simulink model "case2"  (R2024b)
settings: Solver=FixedStepAuto  StartTime=0  StopTime=1  FixedStep=1e-7  RelTol=1e-3
values from neighbouring files (symbols this model uses):
  SG_D_1_D = 0.01056    [IEEE9_case_parameters.m]    (also in case1_parameters.m; case2_parameters.m; case3_parameters.m; case4_parameters.m)
  SG_D_1_EnableSaturation = 0    [IEEE9_case_parameters.m]    (also in case1_parameters.m; case2_parameters.m; case3_parameters.m; case4_parameters.m)
  SG_D_1_f0 = 60    [IEEE9_case_parameters.m]    (also in case1_parameters.m; case2_parameters.m; case3_parameters.m; case4_parameters.m)
  SG_D_1_H = 7.5    [IEEE9_case_parameters.m]    (also in case1_parameters.m; case2_parameters.m; case3_parameters.m; case4_parameters.m)
  SG_D_1_K_A = 20    [IEEE9_case_parameters.m]    (also in case1_parameters.m; case2_parameters.m; case3_parameters.m; case4_parameters.m)
  SG_D_1_K_E = 1.000000e+1    (= 10)    [IEEE9_case_parameters.m]    (also in case1_parameters.m; case2_parameters.m; case3_parameters.m; case4_parameters.m)
  SG_D_1_K_F = 2.363    [IEEE9_case_parameters.m]    (also in case1_parameters.m; case2_parameters.m; case3_parameters.m; case4_parameters.m)
  SG_D_1_K_s = 0.5    [IEEE9_case_parameters.m]    (also in case1_parameters.m = 5; case2_parameters.m = 5; case3_parameters.m = 5; case4_parameters.m = 5)
  SG_D_1_R_a = 0.001088    [IEEE9_case_parameters.m]    (also in case1_parameters.m; case2_parameters.m; case3_parameters.m; case4_parameters.m)
  SG_D_1_S_A = 1    [IEEE9_case_parameters.m]    (also in case1_parameters.m; case2_parameters.m; case3_parameters.m; case4_parameters.m)
  SG_D_1_S_B = 0.103    [IEEE9_case_parameters.m]    (also in case1_parameters.m; case2_parameters.m; case3_parameters.m; case4_parameters.m)
  SG_D_1_S_N = 10.659857    [IEEE9_case_parameters.m]    (also in case1_parameters.m; case2_parameters.m; case3_parameters.m; case4_parameters.m)
  SG_D_1_SpeedPara = 200    [IEEE9_case_parameters.m]    (also in case1_parameters.m; case2_parameters.m; case3_parameters.m; case4_parameters.m)
  SG_D_1_T_0 = 0.720173    [IEEE9_case_parameters.m]    (also in case1_parameters.m = 0.755522; case2_parameters.m = 0.808931; case3_parameters.m = 0.869402; case4_parameters.m = 0.729316)
  SG_D_1_T_1 = 0.3    [IEEE9_case_parameters.m]    (also in case1_parameters.m; case2_parameters.m; case3_parameters.m; case4_parameters.m)
  SG_D_1_T_2 = 0.05    [IEEE9_case_parameters.m]    (also in case1_parameters.m; case2_parameters.m; case3_parameters.m; case4_parameters.m)
  SG_D_1_T_3 = 0.02    [IEEE9_case_parameters.m]    (also in case1_parameters.m; case2_parameters.m; case3_parameters.m; case4_parameters.m)
  SG_D_1_T_4 = 0.005    [IEEE9_case_parameters.m]    (also in case1_parameters.m; case2_parameters.m; case3_parameters.m; case4_parameters.m)
  SG_D_1_T_A = 0.02    [IEEE9_case_parameters.m]    (also in case1_parameters.m; case2_parameters.m; case3_parameters.m; case4_parameters.m)
  SG_D_1_T_dd = 8.000000e+0    (= 8)    [IEEE9_case_parameters.m]    (also in case1_parameters.m; case2_parameters.m; case3_parameters.m; case4_parameters.m)
  SG_D_1_T_ddd = 0.04    [IEEE9_case_parameters.m]    (also in case1_parameters.m; case2_parameters.m; case3_parameters.m; case4_parameters.m)
  SG_D_1_T_E = 0.314    [IEEE9_case_parameters.m]    (also in case1_parameters.m; case2_parameters.m; case3_parameters.m; case4_parameters.m)
  SG_D_1_T_F = 0.35    [IEEE9_case_parameters.m]    (also in case1_parameters.m; case2_parameters.m; case3_parameters.m; case4_parameters.m)
  SG_D_1_T_qd = 0.8    [IEEE9_case_parameters.m]    (also in case1_parameters.m; case2_parameters.m; case3_parameters.m; case4_parameters.m)
  SG_D_1_T_qdd = 0.02    [IEEE9_case_parameters.m]    (also in case1_parameters.m; case2_parameters.m; case3_parameters.m; case4_parameters.m)
  SG_D_1_T_speed = 0.1    [IEEE9_case_parameters.m]    (also in case1_parameters.m = 200; case2_parameters.m = 200; case3_parameters.m = 200; case4_parameters.m = 200)
  SG_D_1_T_w = 0.5    [IEEE9_case_parameters.m]    (also in case1_parameters.m; case2_parameters.m; case3_parameters.m; case4_parameters.m)
  SG_D_1_V_ref = 1.990276    [IEEE9_case_parameters.m]    (also in case1_parameters.m = 2.042296; case2_parameters.m = 2.051388; case3_parameters.m = 2.089584; case4_parameters.m = 2.01845)
  SG_D_1_w_ref = 376.991118    [IEEE9_case_parameters.m]    (also in case1_parameters.m; case2_parameters.m; case3_parameters.m; case4_parameters.m)
  SG_D_1_wb = 6.000000e+1    (= 60)    [IEEE9_case_parameters.m]    (also in case1_parameters.m; case2_parameters.m; case3_parameters.m; case4_parameters.m)
  SG_D_1_x_d = 1.9    [IEEE9_case_parameters.m]    (also in case1_parameters.m; case2_parameters.m; case3_parameters.m; case4_parameters.m)
  SG_D_1_x_dd = 0.302    [IEEE9_case_parameters.m]    (also in case1_parameters.m; case2_parameters.m; case3_parameters.m; case4_parameters.m)
  SG_D_1_x_ddd = 0.204    [IEEE9_case_parameters.m]    (also in case1_parameters.m; case2_parameters.m; case3_parameters.m; case4_parameters.m)
  SG_D_1_x_l = 0.05    [IEEE9_case_parameters.m]    (also in case1_parameters.m; case2_parameters.m; case3_parameters.m; case4_parameters.m)
  SG_D_1_x_q = 1.3    [IEEE9_case_parameters.m]    (also in case1_parameters.m; case2_parameters.m; case3_parameters.m; case4_parameters.m)
  SG_D_1_x_qd = 0.5    [IEEE9_case_parameters.m]    (also in case1_parameters.m; case2_parameters.m; case3_parameters.m; case4_parameters.m)
  SG_D_1_x_qdd = 0.3    [IEEE9_case_parameters.m]    (also in case1_parameters.m; case2_parameters.m; case3_parameters.m; case4_parameters.m)
  SG_D_2_D = 0.02    [IEEE9_case_parameters.m]    (also in case1_parameters.m; case2_parameters.m; case3_parameters.m; case4_parameters.m)
  SG_D_2_EnableSaturation = 0    [IEEE9_case_parameters.m]    (also in case1_parameters.m; case2_parameters.m; case3_parameters.m; case4_parameters.m)
  SG_D_2_f0 = 60    [IEEE9_case_parameters.m]    (also in case1_parameters.m; case2_parameters.m; case3_parameters.m; case4_parameters.m)
  SG_D_2_H = 8.000000e+0    (= 8)    [IEEE9_case_parameters.m]    (also in case1_parameters.m; case2_parameters.m; case3_parameters.m; case4_parameters.m)
  SG_D_2_K_A = 20    [IEEE9_case_parameters.m]    (also in case1_parameters.m; case2_parameters.m; case3_parameters.m; case4_parameters.m)
  SG_D_2_K_E = 1.000000e+1    (= 10)    [IEEE9_case_parameters.m]    (also in case1_parameters.m; case2_parameters.m; case3_parameters.m; case4_parameters.m)
  SG_D_2_K_F = 2.363    [IEEE9_case_parameters.m]    (also in case1_parameters.m; case2_parameters.m; case3_parameters.m; case4_parameters.m)
  SG_D_2_K_s = 0.5    [IEEE9_case_parameters.m]    (also in case1_parameters.m = 4; case2_parameters.m = 4; case3_parameters.m = 4; case4_parameters.m = 4)
  SG_D_2_R_a = 0.001088    [IEEE9_case_parameters.m]    (also in case1_parameters.m; case2_parameters.m; case3_parameters.m; case4_parameters.m)
  SG_D_2_S_A = 1    [IEEE9_case_parameters.m]    (also in case1_parameters.m; case2_parameters.m; case3_parameters.m; case4_parameters.m)
  SG_D_2_S_B = 0.103    [IEEE9_case_parameters.m]    (also in case1_parameters.m; case2_parameters.m; case3_parameters.m; case4_parameters.m)
  SG_D_2_S_N = 10.659857    [IEEE9_case_parameters.m]    (also in case1_parameters.m; case2_parameters.m; case3_parameters.m; case4_parameters.m)
  SG_D_2_SpeedPara = 200    [IEEE9_case_parameters.m]    (also in case1_parameters.m; case2_parameters.m; case3_parameters.m; case4_parameters.m)
  SG_D_2_T_0 = 1.632913    [IEEE9_case_parameters.m]    (also in case1_parameters.m = 1.632925; case2_parameters.m = 1.632915; case3_parameters.m = 1.632914; case4_parameters.m = 1.632927)
  SG_D_2_T_1 = 0.2    [IEEE9_case_parameters.m]    (also in case1_parameters.m; case2_parameters.m; case3_parameters.m; case4_parameters.m)
  SG_D_2_T_2 = 0.05    [IEEE9_case_parameters.m]    (also in case1_parameters.m; case2_parameters.m; case3_parameters.m; case4_parameters.m)
  SG_D_2_T_3 = 0.02    [IEEE9_case_parameters.m]    (also in case1_parameters.m; case2_parameters.m; case3_parameters.m; case4_parameters.m)
  SG_D_2_T_4 = 0.005    [IEEE9_case_parameters.m]    (also in case1_parameters.m; case2_parameters.m; case3_parameters.m; case4_parameters.m)
  SG_D_2_T_A = 0.02    [IEEE9_case_parameters.m]    (also in case1_parameters.m; case2_parameters.m; case3_parameters.m; case4_parameters.m)
  SG_D_2_T_dd = 7.9    [IEEE9_case_parameters.m]    (also in case1_parameters.m; case2_parameters.m; case3_parameters.m; case4_parameters.m)
  SG_D_2_T_ddd = 0.04    [IEEE9_case_parameters.m]    (also in case1_parameters.m; case2_parameters.m; case3_parameters.m; case4_parameters.m)
  SG_D_2_T_E = 0.314    [IEEE9_case_parameters.m]    (also in case1_parameters.m; case2_parameters.m; case3_parameters.m; case4_parameters.m)
  SG_D_2_T_F = 0.35    [IEEE9_case_parameters.m]    (also in case1_parameters.m; case2_parameters.m; case3_parameters.m; case4_parameters.m)
  SG_D_2_T_qd = 0.8    [IEEE9_case_parameters.m]    (also in case1_parameters.m; case2_parameters.m; case3_parameters.m; case4_parameters.m)
  SG_D_2_T_qdd = 0.015    [IEEE9_case_parameters.m]    (also in case1_parameters.m; case2_parameters.m; case3_parameters.m; case4_parameters.m)
  SG_D_2_T_speed = 0.1    [IEEE9_case_parameters.m]    (also in case1_parameters.m = 150; case2_parameters.m = 150; case3_parameters.m = 150; case4_parameters.m = 150)
  SG_D_2_T_w = 0.35    [IEEE9_case_parameters.m]    (also in case1_parameters.m; case2_parameters.m; case3_parameters.m; case4_parameters.m)
  SG_D_2_V_ref = 2.58547    [IEEE9_case_parameters.m]    (also in case1_parameters.m = 2.597896; case2_parameters.m = 2.587136; case3_parameters.m = 2.586042; case4_parameters.m = 2.599679)
  SG_D_2_w_ref = 376.991118    [IEEE9_case_parameters.m]    (also in case1_parameters.m; case2_parameters.m; case3_parameters.m; case4_parameters.m)
  SG_D_2_wb = 6.000000e+1    (= 60)    [IEEE9_case_parameters.m]    (also in case1_parameters.m; case2_parameters.m; case3_parameters.m; case4_parameters.m)
  SG_D_2_x_d = 1.8    [IEEE9_case_parameters.m]    (also in case1_parameters.m; case2_parameters.m; case3_parameters.m; case4_parameters.m)
  SG_D_2_x_dd = 0.302    [IEEE9_case_parameters.m]    (also in case1_parameters.m; case2_parameters.m; case3_parameters.m; case4_parameters.m)
  SG_D_2_x_ddd = 0.204    [IEEE9_case_parameters.m]    (also in case1_parameters.m; case2_parameters.m; case3_parameters.m; case4_parameters.m)
  SG_D_2_x_l = 0.05    [IEEE9_case_parameters.m]    (also in case1_parameters.m; case2_parameters.m; case3_parameters.m; case4_parameters.m)
  SG_D_2_x_q = 1.25    [IEEE9_case_parameters.m]    (also in case1_parameters.m; case2_parameters.m; case3_parameters.m; case4_parameters.m)
  SG_D_2_x_qd = 0.5    [IEEE9_case_parameters.m]    (also in case1_parameters.m; case2_parameters.m; case3_parameters.m; case4_parameters.m)
  SG_D_2_x_qdd = 0.3    [IEEE9_case_parameters.m]    (also in case1_parameters.m; case2_parameters.m; case3_parameters.m; case4_parameters.m)
  SG_D_3_D = 0.02    [IEEE9_case_parameters.m]    (also in case1_parameters.m; case2_parameters.m; case3_parameters.m; case4_parameters.m)
  SG_D_3_EnableSaturation = 0    [IEEE9_case_parameters.m]    (also in case1_parameters.m; case2_parameters.m; case3_parameters.m; case4_parameters.m)
  SG_D_3_f0 = 60    [IEEE9_case_parameters.m]    (also in case1_parameters.m; case2_parameters.m; case3_parameters.m; case4_parameters.m)
  SG_D_3_H = 7.7    [IEEE9_case_parameters.m]    (also in case1_parameters.m; case2_parameters.m; case3_parameters.m; case4_parameters.m)
  SG_D_3_K_A = 20    [IEEE9_case_parameters.m]    (also in case1_parameters.m; case2_parameters.m; case3_parameters.m; case4_parameters.m)
  SG_D_3_K_E = 1.000000e+1    (= 10)    [IEEE9_case_parameters.m]    (also in case1_parameters.m; case2_parameters.m; case3_parameters.m; case4_parameters.m)
  SG_D_3_K_F = 2.363    [IEEE9_case_parameters.m]    (also in case1_parameters.m; case2_parameters.m; case3_parameters.m; case4_parameters.m)
  SG_D_3_K_s = 0.2    [IEEE9_case_parameters.m]    (also in case1_parameters.m = 2; case2_parameters.m = 2; case3_parameters.m = 2; case4_parameters.m = 2)
  SG_D_3_R_a = 0.001088    [IEEE9_case_parameters.m]    (also in case1_parameters.m; case2_parameters.m; case3_parameters.m; case4_parameters.m)
  SG_D_3_S_A = 1    [IEEE9_case_parameters.m]    (also in case1_parameters.m; case2_parameters.m; case3_parameters.m; case4_parameters.m)
  SG_D_3_S_B = 0.103    [IEEE9_case_parameters.m]    (also in case1_parameters.m; case2_parameters.m; case3_parameters.m; case4_parameters.m)
  SG_D_3_S_N = 10.659857    [IEEE9_case_parameters.m]    (also in case1_parameters.m; case2_parameters.m; case3_parameters.m; case4_parameters.m)
  SG_D_3_SpeedPara = 200    [IEEE9_case_parameters.m]    (also in case1_parameters.m; case2_parameters.m; case3_parameters.m; case4_parameters.m)
  SG_D_3_T_0 = 0.850788    [IEEE9_case_parameters.m]    (also in case1_parameters.m = 0.850786; case2_parameters.m = 0.850787; case3_parameters.m; case4_parameters.m = 0.850786)
  SG_D_3_T_1 = 0.2    [IEEE9_case_parameters.m]    (also in case1_parameters.m; case2_parameters.m; case3_parameters.m; case4_parameters.m)
  SG_D_3_T_2 = 0.05    [IEEE9_case_parameters.m]    (also in case1_parameters.m; case2_parameters.m; case3_parameters.m; case4_parameters.m)
  SG_D_3_T_3 = 0.02    [IEEE9_case_parameters.m]    (also in case1_parameters.m; case2_parameters.m; case3_parameters.m; case4_parameters.m)
  SG_D_3_T_4 = 0.005    [IEEE9_case_parameters.m]    (also in case1_parameters.m; case2_parameters.m; case3_parameters.m; case4_parameters.m)
  SG_D_3_T_A = 0.02    [IEEE9_case_parameters.m]    (also in case1_parameters.m; case2_parameters.m; case3_parameters.m; case4_parameters.m)
  SG_D_3_T_dd = 8.1    [IEEE9_case_parameters.m]    (also in case1_parameters.m; case2_parameters.m; case3_parameters.m; case4_parameters.m)
  SG_D_3_T_ddd = 0.04    [IEEE9_case_parameters.m]    (also in case1_parameters.m; case2_parameters.m; case3_parameters.m; case4_parameters.m)
  SG_D_3_T_E = 0.314    [IEEE9_case_parameters.m]    (also in case1_parameters.m; case2_parameters.m; case3_parameters.m; case4_parameters.m)
  SG_D_3_T_F = 0.35    [IEEE9_case_parameters.m]    (also in case1_parameters.m; case2_parameters.m; case3_parameters.m; case4_parameters.m)
  SG_D_3_T_qd = 0.8    [IEEE9_case_parameters.m]    (also in case1_parameters.m; case2_parameters.m; case3_parameters.m; case4_parameters.m)
  SG_D_3_T_qdd = 0.015    [IEEE9_case_parameters.m]    (also in case1_parameters.m; case2_parameters.m; case3_parameters.m; case4_parameters.m)
  SG_D_3_T_speed = 0.1    [IEEE9_case_parameters.m]    (also in case1_parameters.m = 180; case2_parameters.m = 180; case3_parameters.m = 180; case4_parameters.m = 180)
  SG_D_3_T_w = 0.4    [IEEE9_case_parameters.m]    (also in case1_parameters.m; case2_parameters.m; case3_parameters.m; case4_parameters.m)
  SG_D_3_V_ref = 1.892727    [IEEE9_case_parameters.m]    (also in case1_parameters.m = 1.906439; case2_parameters.m = 1.895535; case3_parameters.m = 1.892105; case4_parameters.m = 1.906598)
  SG_D_3_w_ref = 376.991118    [IEEE9_case_parameters.m]    (also in case1_parameters.m; case2_parameters.m; case3_parameters.m; case4_parameters.m)
  SG_D_3_wb = 6.000000e+1    (= 60)    [IEEE9_case_parameters.m]    (also in case1_parameters.m; case2_parameters.m; case3_parameters.m; case4_parameters.m)
  SG_D_3_x_d = 1.85    [IEEE9_case_parameters.m]    (also in case1_parameters.m; case2_parameters.m; case3_parameters.m; case4_parameters.m)
  SG_D_3_x_dd = 0.302    [IEEE9_case_parameters.m]    (also in case1_parameters.m; case2_parameters.m; case3_parameters.m; case4_parameters.m)
  SG_D_3_x_ddd = 0.204    [IEEE9_case_parameters.m]    (also in case1_parameters.m; case2_parameters.m; case3_parameters.m; case4_parameters.m)
  SG_D_3_x_l = 0.05    [IEEE9_case_parameters.m]    (also in case1_parameters.m; case2_parameters.m; case3_parameters.m; case4_parameters.m)
  SG_D_3_x_q = 1.2    [IEEE9_case_parameters.m]    (also in case1_parameters.m; case2_parameters.m; case3_parameters.m; case4_parameters.m)
  SG_D_3_x_qd = 0.5    [IEEE9_case_parameters.m]    (also in case1_parameters.m; case2_parameters.m; case3_parameters.m; case4_parameters.m)
  SG_D_3_x_qdd = 0.3    [IEEE9_case_parameters.m]    (also in case1_parameters.m; case2_parameters.m; case3_parameters.m; case4_parameters.m)
(part 2 of 12)

== system case2/SG_D_2 ==
  v_d_SG_D_2 : Inport
  v_q_SG_D_2 : Inport  Port=2
  E_fd_SG_D_2 : Integrator  InitialCondition=3.174272760835506
  Px_1_SG_D_2 : Integrator  InitialCondition=0.0
  Px_2_SG_D_2 : Integrator  InitialCondition=0.0
  Px_3_SG_D_2 : Integrator  InitialCondition=1.5518206865207427e-24
  R_f_SG_D_2 : Integrator  InitialCondition=21.43087581101229
  T_e_SG_D_2_block : Subsystem
  T_m_SG_D_2 : Integrator  InitialCondition=1.6329149167652506
  V_f_SG_D_2 : Integrator  InitialCondition=31.742727608355057
  d_E_fd_SG_D_2_block : Subsystem
  d_Px_1_SG_D_2_block : Subsystem
  d_Px_2_SG_D_2_block : Subsystem
  d_Px_3_SG_D_2_block : Subsystem
  d_R_f_SG_D_2_block : Subsystem
  d_T_m_SG_D_2_block : Subsystem
  d_V_f_SG_D_2_block : Subsystem
  d_psi_1d_SG_D_2_block : Subsystem
  d_psi_d_SG_D_2_block : Subsystem
  d_psi_fd_SG_D_2_block : Subsystem
  d_psi_gq_SG_D_2_block : Subsystem
  d_psi_kq_SG_D_2_block : Subsystem
  d_psi_q_SG_D_2_block : Subsystem
  d_theta_SG_D_2_block : Subsystem
  d_w_SG_D_2_block : Subsystem
  i_d_SG_D_2_block : Subsystem
  i_q_SG_D_2_block : Subsystem
  psi_1d_SG_D_2 : Integrator  InitialCondition=0.5787158687798319
  psi_d_SG_D_2 : Integrator  InitialCondition=0.504557100435384
  psi_fd_SG_D_2 : Integrator  InitialCondition=0.9524760612358489
  psi_gq_SG_D_2 : Integrator  InitialCondition=0.5192590741580433
  psi_kq_SG_D_2 : Integrator  InitialCondition=-0.8308145186528693
  psi_q_SG_D_2 : Integrator  InitialCondition=-0.8654317902634056
  theta_SG_D_2 : Integrator  InitialCondition=1.1962684178296192
  theta_SG_D_2_out_block : Subsystem
  w_SG_D_2 : Integrator  InitialCondition=376.99111843077515
  w_SG_D_2_out_block : Subsystem
  i_d_SG_D_2 : Outport
  i_q_SG_D_2 : Outport  Port=2
  T_e_SG_D_2 : Outport  Port=3
  w_SG_D_2_out : Outport  Port=4
  theta_SG_D_2_out : Outport  Port=5
  wires:
  d_T_m_SG_D_2_block/1(Blockout_d_T_m_SG_D_2_4b089) -> T_m_SG_D_2/1
  T_e_SG_D_2_block/1(Blockout_T_e_SG_D_2_b8deb) -> T_e_SG_D_2/1
  d_Px_2_SG_D_2_block/1(Blockout_d_Px_2_SG_D_2_22689) -> Px_2_SG_D_2/1
  w_SG_D_2/1 -> d_psi_d_SG_D_2_block/9(State_w_SG_D_2_e892d), d_w_SG_D_2_block/1(State_w_SG_D_2_a0af8), d_V_f_SG_D_2_block/13(State_w_SG_D_2_f97cf), d_psi_q_SG_D_2_block/9(State_w_SG_D_2_c2d17), d_V_f_SG_D_2_block/8(State_w_SG_D_2_9712b), d_theta_SG_D_2_block/1(State_w_SG_D_2_08923), d_Px_2_SG_D_2_block/4(State_w_SG_D_2_45781), d_Px_3_SG_D_2_block/6(State_w_SG_D_2_38541), d_Px_1_SG_D_2_block/2(State_w_SG_D_2_84017), w_SG_D_2_out_block/1(State_w_SG_D_2_b0f95), d_T_m_SG_D_2_block/1(State_w_SG_D_2_14e8c)
  d_theta_SG_D_2_block/1(Blockout_d_theta_SG_D_2_633fd) -> theta_SG_D_2/1
  d_Px_1_SG_D_2_block/1(Blockout_d_Px_1_SG_D_2_b8a6d) -> Px_1_SG_D_2/1
  psi_q_SG_D_2/1 -> d_psi_d_SG_D_2_block/8(State_psi_q_SG_D_2_fe7e7), d_psi_q_SG_D_2_block/3(State_psi_q_SG_D_2_bc55a), d_psi_gq_SG_D_2_block/6(State_psi_q_SG_D_2_40973), d_psi_gq_SG_D_2_block/9(State_psi_q_SG_D_2_4a342), d_psi_kq_SG_D_2_block/5(State_psi_q_SG_D_2_76d71), d_w_SG_D_2_block/7(State_psi_q_SG_D_2_3518a), d_V_f_SG_D_2_block/7(State_psi_q_SG_D_2_f4c0e), d_w_SG_D_2_block/6(State_psi_q_SG_D_2_c02e1), d_V_f_SG_D_2_block/11(State_psi_q_SG_D_2_6c1aa), i_q_SG_D_2_block/3(State_psi_q_SG_D_2_d1f7c), i_d_SG_D_2_block/3(State_psi_q_SG_D_2_74918), T_e_SG_D_2_block/4(State_psi_q_SG_D_2_d45b5), T_e_SG_D_2_block/5(State_psi_q_SG_D_2_80989)
  w_SG_D_2_out_block/1(Blockout_w_SG_D_2_out_f6fd7) -> w_SG_D_2_out/1
  psi_fd_SG_D_2/1 -> d_psi_fd_SG_D_2_block/2(State_psi_fd_SG_D_2_9a5f7), d_psi_fd_SG_D_2_block/4(State_psi_fd_SG_D_2_7d5d1), d_psi_1d_SG_D_2_block/2(State_psi_fd_SG_D_2_21e47), d_V_f_SG_D_2_block/6(State_psi_fd_SG_D_2_145b7), d_w_SG_D_2_block/10(State_psi_fd_SG_D_2_89ccd), T_e_SG_D_2_block/8(State_psi_fd_SG_D_2_cd007), d_psi_fd_SG_D_2_block/7(State_psi_fd_SG_D_2_aa5d6), i_q_SG_D_2_block/7(State_psi_fd_SG_D_2_212cc), i_d_SG_D_2_block/7(State_psi_fd_SG_D_2_463f2), d_psi_1d_SG_D_2_block/5(State_psi_fd_SG_D_2_221ae), d_psi_d_SG_D_2_block/3(State_psi_fd_SG_D_2_19126), d_psi_fd_SG_D_2_block/10(State_psi_fd_SG_D_2_e8112)
  d_Px_3_SG_D_2_block/1(Blockout_d_Px_3_SG_D_2_0a542) -> Px_3_SG_D_2/1
  v_d_SG_D_2/1 -> d_psi_d_SG_D_2_block/4(Input_v_d_SG_D_2_3ae72), d_psi_q_SG_D_2_block/4(Input_v_d_SG_D_2_0f316)
  d_V_f_SG_D_2_block/1(Blockout_d_V_f_SG_D_2_fa732) -> V_f_SG_D_2/1
  v_q_SG_D_2/1 -> d_psi_d_SG_D_2_block/6(Input_v_q_SG_D_2_cabf7), d_psi_q_SG_D_2_block/6(Input_v_q_SG_D_2_6312d)
  theta_SG_D_2/1 -> i_d_SG_D_2_block/4(State_theta_SG_D_2_67c6e), d_psi_q_SG_D_2_block/5(State_theta_SG_D_2_f78f2), d_psi_d_SG_D_2_block/7(State_theta_SG_D_2_a0973), i_d_SG_D_2_block/8(State_theta_SG_D_2_e4d3c), d_psi_d_SG_D_2_block/5(State_theta_SG_D_2_01400), d_psi_q_SG_D_2_block/7(State_theta_SG_D_2_25da5), i_q_SG_D_2_block/8(State_theta_SG_D_2_6d11f), theta_SG_D_2_out_block/1(State_theta_SG_D_2_6b056), i_q_SG_D_2_block/4(State_theta_SG_D_2_14f06)
  Px_2_SG_D_2/1 -> d_Px_3_SG_D_2_block/2(State_Px_2_SG_D_2_61639), d_Px_3_SG_D_2_block/3(State_Px_2_SG_D_2_4e1b7), d_Px_2_SG_D_2_block/1(State_Px_2_SG_D_2_f980a)
  psi_gq_SG_D_2/1 -> d_psi_q_SG_D_2_block/1(State_psi_gq_SG_D_2_02402), d_psi_gq_SG_D_2_block/1(State_psi_gq_SG_D_2_a2a06), d_psi_gq_SG_D_2_block/2(State_psi_gq_SG_D_2_83ab1), d_psi_gq_SG_D_2_block/4(State_psi_gq_SG_D_2_c1c72), d_psi_kq_SG_D_2_block/1(State_psi_gq_SG_D_2_2ecc4), d_psi_kq_SG_D_2_block/3(State_psi_gq_SG_D_2_6238c), d_V_f_SG_D_2_block/9(State_psi_gq_SG_D_2_6385a), d_psi_gq_SG_D_2_block/7(State_psi_gq_SG_D_2_7b31f), i_q_SG_D_2_block/1(State_psi_gq_SG_D_2_62065), d_w_SG_D_2_block/4(State_psi_gq_SG_D_2_fa13f), T_e_SG_D_2_block/2(State_psi_gq_SG_D_2_708b9), i_d_SG_D_2_block/1(State_psi_gq_SG_D_2_419a5)
  psi_1d_SG_D_2/1 -> d_psi_fd_SG_D_2_block/3(State_psi_1d_SG_D_2_9e249), d_psi_fd_SG_D_2_block/8(State_psi_1d_SG_D_2_c9b22), d_psi_fd_SG_D_2_block/5(State_psi_1d_SG_D_2_19e55), d_psi_d_SG_D_2_block/1(State_psi_1d_SG_D_2_3fdee), d_psi_1d_SG_D_2_block/1(State_psi_1d_SG_D_2_7ee43), d_psi_1d_SG_D_2_block/3(State_psi_1d_SG_D_2_6e6f3), d_w_SG_D_2_block/8(State_psi_1d_SG_D_2_8aa3a), d_V_f_SG_D_2_block/4(State_psi_1d_SG_D_2_c0128), i_d_SG_D_2_block/5(State_psi_1d_SG_D_2_37338), i_q_SG_D_2_block/5(State_psi_1d_SG_D_2_3e03a), T_e_SG_D_2_block/6(State_psi_1d_SG_D_2_98cfc)
  T_m_SG_D_2/1 -> d_T_m_SG_D_2_block/2(State_T_m_SG_D_2_165ac), d_w_SG_D_2_block/2(State_T_m_SG_D_2_deb70)
  Px_1_SG_D_2/1 -> d_Px_1_SG_D_2_block/1(State_Px_1_SG_D_2_d590c), d_Px_3_SG_D_2_block/4(State_Px_1_SG_D_2_cef04), d_Px_3_SG_D_2_block/5(State_Px_1_SG_D_2_2a306), d_Px_2_SG_D_2_block/3(State_Px_1_SG_D_2_9c84f), d_Px_2_SG_D_2_block/2(State_Px_1_SG_D_2_3257e)
  i_d_SG_D_2_block/1(Blockout_i_d_SG_D_2_4df8b) -> i_d_SG_D_2/1
  psi_d_SG_D_2/1 -> d_psi_fd_SG_D_2_block/6(State_psi_d_SG_D_2_bc679), d_psi_fd_SG_D_2_block/9(State_psi_d_SG_D_2_749a1), d_psi_d_SG_D_2_block/2(State_psi_d_SG_D_2_d60ed), d_psi_q_SG_D_2_block/8(State_psi_d_SG_D_2_afeb6), d_psi_1d_SG_D_2_block/4(State_psi_d_SG_D_2_2e599), d_w_SG_D_2_block/3(State_psi_d_SG_D_2_6bbdf), d_V_f_SG_D_2_block/12(State_psi_d_SG_D_2_bc1e6), i_d_SG_D_2_block/6(State_psi_d_SG_D_2_8c17d), i_q_SG_D_2_block/6(State_psi_d_SG_D_2_1a46c), d_w_SG_D_2_block/9(State_psi_d_SG_D_2_a921b), T_e_SG_D_2_block/1(State_psi_d_SG_D_2_1b998), T_e_SG_D_2_block/7(State_psi_d_SG_D_2_92f27), d_V_f_SG_D_2_block/5(State_psi_d_SG_D_2_b5e07)
  psi_kq_SG_D_2/1 -> d_psi_q_SG_D_2_block/2(State_psi_kq_SG_D_2_3ae4e), d_psi_gq_SG_D_2_block/5(State_psi_kq_SG_D_2_816be), d_psi_kq_SG_D_2_block/2(State_psi_kq_SG_D_2_ff9b7), d_psi_kq_SG_D_2_block/4(State_psi_kq_SG_D_2_b8096), d_w_SG_D_2_block/5(State_psi_kq_SG_D_2_e86be), d_V_f_SG_D_2_block/10(State_psi_kq_SG_D_2_aa54e), i_q_SG_D_2_block/2(State_psi_kq_SG_D_2_46994), T_e_SG_D_2_block/3(State_psi_kq_SG_D_2_15175), d_psi_gq_SG_D_2_block/3(State_psi_kq_SG_D_2_ccf89), i_d_SG_D_2_block/2(State_psi_kq_SG_D_2_2885e), d_psi_gq_SG_D_2_block/8(State_psi_kq_SG_D_2_a9de5)
  d_psi_1d_SG_D_2_block/1(Blockout_d_psi_1d_SG_D_2_52177) -> psi_1d_SG_D_2/1
  d_psi_q_SG_D_2_block/1(Blockout_d_psi_q_SG_D_2_71529) -> psi_q_SG_D_2/1
  d_psi_d_SG_D_2_block/1(Blockout_d_psi_d_SG_D_2_b24b5) -> psi_d_SG_D_2/1
  d_psi_kq_SG_D_2_block/1(Blockout_d_psi_kq_SG_D_2_e0637) -> psi_kq_SG_D_2/1
  i_q_SG_D_2_block/1(Blockout_i_q_SG_D_2_bbd87) -> i_q_SG_D_2/1
  R_f_SG_D_2/1 -> d_R_f_SG_D_2_block/2(State_R_f_SG_D_2_5b4f1), d_V_f_SG_D_2_block/2(State_R_f_SG_D_2_7d620)
  theta_SG_D_2_out_block/1(Blockout_theta_SG_D_2_out_ba39c) -> theta_SG_D_2_out/1
  d_w_SG_D_2_block/1(Blockout_d_w_SG_D_2_da6a7) -> w_SG_D_2/1
  d_psi_gq_SG_D_2_block/1(Blockout_d_psi_gq_SG_D_2_be7cc) -> psi_gq_SG_D_2/1
  d_R_f_SG_D_2_block/1(Blockout_d_R_f_SG_D_2_fdb54) -> R_f_SG_D_2/1
  V_f_SG_D_2/1 -> d_V_f_SG_D_2_block/14(State_V_f_SG_D_2_2e53e), d_E_fd_SG_D_2_block/2(State_V_f_SG_D_2_edff6)
  Px_3_SG_D_2/1 -> d_Px_3_SG_D_2_block/1(State_Px_3_SG_D_2_650ae), d_V_f_SG_D_2_block/3(State_Px_3_SG_D_2_fb941)
  d_E_fd_SG_D_2_block/1(Blockout_d_E_fd_SG_D_2_d404e) -> E_fd_SG_D_2/1
  E_fd_SG_D_2/1 -> d_V_f_SG_D_2_block/1(State_E_fd_SG_D_2_39bcd), d_R_f_SG_D_2_block/1(State_E_fd_SG_D_2_001ad), d_E_fd_SG_D_2_block/1(State_E_fd_SG_D_2_04f17), d_psi_fd_SG_D_2_block/1(State_E_fd_SG_D_2_538cb)
  d_psi_fd_SG_D_2_block/1(Blockout_d_psi_fd_SG_D_2_3c09c) -> psi_fd_SG_D_2/1

== system case2/SG_D_3 ==
  v_d_SG_D_3 : Inport
  v_q_SG_D_3 : Inport  Port=2
  E_fd_SG_D_3 : Integrator  InitialCondition=1.7910701006182943
  Px_1_SG_D_3 : Integrator  InitialCondition=0.0
  Px_2_SG_D_3 : Integrator  InitialCondition=0.0
  Px_3_SG_D_3 : Integrator  InitialCondition=-1.0387374102072241e-24
  R_f_SG_D_3 : Integrator  InitialCondition=12.092281850745799
  T_e_SG_D_3_block : Subsystem
  T_m_SG_D_3 : Integrator  InitialCondition=0.8507871254664061
  V_f_SG_D_3 : Integrator  InitialCondition=17.910701006182943
  d_E_fd_SG_D_3_block : Subsystem
  d_Px_1_SG_D_3_block : Subsystem
  d_Px_2_SG_D_3_block : Subsystem
  d_Px_3_SG_D_3_block : Subsystem
  d_R_f_SG_D_3_block : Subsystem
  d_T_m_SG_D_3_block : Subsystem
  d_V_f_SG_D_3_block : Subsystem
  d_psi_1d_SG_D_3_block : Subsystem
  d_psi_d_SG_D_3_block : Subsystem
  d_psi_fd_SG_D_3_block : Subsystem
  d_psi_gq_SG_D_3_block : Subsystem
  d_psi_kq_SG_D_3_block : Subsystem
  d_psi_q_SG_D_3_block : Subsystem
  d_theta_SG_D_3_block : Subsystem
  d_w_SG_D_3_block : Subsystem
  i_d_SG_D_3_block : Subsystem
  i_q_SG_D_3_block : Subsystem
  psi_1d_SG_D_3 : Integrator  InitialCondition=0.7172513618057285
  psi_d_SG_D_3 : Integrator  InitialCondition=0.6874230635053793
  psi_fd_SG_D_3 : Integrator  InitialCondition=0.8675859852394877
  psi_gq_SG_D_3 : Integrator  InitialCondition=0.42439253500886276
  psi_kq_SG_D_3 : Integrator  InitialCondition=-0.6972163075145603
  psi_q_SG_D_3 : Integrator  InitialCondition=-0.7275300600151934
  theta_SG_D_3 : Integrator  InitialCondition=0.8839403378010618
  theta_SG_D_3_out_block : Subsystem
  w_SG_D_3 : Integrator  InitialCondition=376.99111843077515
  w_SG_D_3_out_block : Subsystem
  i_d_SG_D_3 : Outport
  i_q_SG_D_3 : Outport  Port=2
  T_e_SG_D_3 : Outport  Port=3
  w_SG_D_3_out : Outport  Port=4
  theta_SG_D_3_out : Outport  Port=5
  wires:
  d_Px_1_SG_D_3_block/1(Blockout_d_Px_1_SG_D_3_ecaac) -> Px_1_SG_D_3/1
  w_SG_D_3/1 -> d_psi_q_SG_D_3_block/9(State_w_SG_D_3_6302a), d_psi_d_SG_D_3_block/9(State_w_SG_D_3_819b4), d_w_SG_D_3_block/1(State_w_SG_D_3_97bb8), d_V_f_SG_D_3_block/8(State_w_SG_D_3_a95f7), d_V_f_SG_D_3_block/13(State_w_SG_D_3_43b52), d_theta_SG_D_3_block/1(State_w_SG_D_3_3d54c), d_T_m_SG_D_3_block/1(State_w_SG_D_3_ad955), d_Px_1_SG_D_3_block/2(State_w_SG_D_3_fb455), d_Px_3_SG_D_3_block/6(State_w_SG_D_3_a9ec3), d_Px_2_SG_D_3_block/4(State_w_SG_D_3_9f660), w_SG_D_3_out_block/1(State_w_SG_D_3_99a7f)
  R_f_SG_D_3/1 -> d_V_f_SG_D_3_block/2(State_R_f_SG_D_3_88428), d_R_f_SG_D_3_block/2(State_R_f_SG_D_3_e823d)
  w_SG_D_3_out_block/1(Blockout_w_SG_D_3_out_0217d) -> w_SG_D_3_out/1
  d_Px_2_SG_D_3_block/1(Blockout_d_Px_2_SG_D_3_b7721) -> Px_2_SG_D_3/1
  d_w_SG_D_3_block/1(Blockout_d_w_SG_D_3_1b2eb) -> w_SG_D_3/1
  Px_1_SG_D_3/1 -> d_Px_1_SG_D_3_block/1(State_Px_1_SG_D_3_6a762), d_Px_3_SG_D_3_block/4(State_Px_1_SG_D_3_dfdda), d_Px_2_SG_D_3_block/3(State_Px_1_SG_D_3_de3ab), d_Px_3_SG_D_3_block/5(State_Px_1_SG_D_3_46ef9), d_Px_2_SG_D_3_block/2(State_Px_1_SG_D_3_07a77)
  d_theta_SG_D_3_block/1(Blockout_d_theta_SG_D_3_7f2c9) -> theta_SG_D_3/1
  d_T_m_SG_D_3_block/1(Blockout_d_T_m_SG_D_3_4be0a) -> T_m_SG_D_3/1
  psi_fd_SG_D_3/1 -> d_psi_fd_SG_D_3_block/2(State_psi_fd_SG_D_3_11ef0), d_psi_fd_SG_D_3_block/4(State_psi_fd_SG_D_3_d3ee5), d_psi_fd_SG_D_3_block/7(State_psi_fd_SG_D_3_7f5a7), d_psi_fd_SG_D_3_block/10(State_psi_fd_SG_D_3_791d9), d_psi_d_SG_D_3_block/3(State_psi_fd_SG_D_3_c348d), d_psi_1d_SG_D_3_block/2(State_psi_fd_SG_D_3_ea669), d_psi_1d_SG_D_3_block/5(State_psi_fd_SG_D_3_4d32c), d_w_SG_D_3_block/10(State_psi_fd_SG_D_3_99c58), d_V_f_SG_D_3_block/6(State_psi_fd_SG_D_3_9c647), i_d_SG_D_3_block/7(State_psi_fd_SG_D_3_d8144), T_e_SG_D_3_block/8(State_psi_fd_SG_D_3_e25ec), i_q_SG_D_3_block/7(State_psi_fd_SG_D_3_16b63)
  d_Px_3_SG_D_3_block/1(Blockout_d_Px_3_SG_D_3_317cb) -> Px_3_SG_D_3/1
  v_d_SG_D_3/1 -> d_psi_d_SG_D_3_block/4(Input_v_d_SG_D_3_4a6e0), d_psi_q_SG_D_3_block/4(Input_v_d_SG_D_3_18c9f)
  v_q_SG_D_3/1 -> d_psi_q_SG_D_3_block/6(Input_v_q_SG_D_3_33c03), d_psi_d_SG_D_3_block/6(Input_v_q_SG_D_3_b307b)
  theta_SG_D_3/1 -> d_psi_d_SG_D_3_block/5(State_theta_SG_D_3_26889), i_q_SG_D_3_block/4(State_theta_SG_D_3_d6326), i_d_SG_D_3_block/4(State_theta_SG_D_3_a77c5), i_d_SG_D_3_block/8(State_theta_SG_D_3_da351), d_psi_q_SG_D_3_block/7(State_theta_SG_D_3_49b48), d_psi_d_SG_D_3_block/7(State_theta_SG_D_3_a755b), i_q_SG_D_3_block/8(State_theta_SG_D_3_67ddf), theta_SG_D_3_out_block/1(State_theta_SG_D_3_32087), d_psi_q_SG_D_3_block/5(State_theta_SG_D_3_06d3e)
  psi_gq_SG_D_3/1 -> d_psi_q_SG_D_3_block/1(State_psi_gq_SG_D_3_520bc), d_psi_gq_SG_D_3_block/4(State_psi_gq_SG_D_3_a44eb), d_psi_gq_SG_D_3_block/1(State_psi_gq_SG_D_3_621ad), d_w_SG_D_3_block/4(State_psi_gq_SG_D_3_6c331), d_psi_gq_SG_D_3_block/7(State_psi_gq_SG_D_3_1d830), d_V_f_SG_D_3_block/9(State_psi_gq_SG_D_3_26e2a), i_d_SG_D_3_block/1(State_psi_gq_SG_D_3_d77e8), d_psi_gq_SG_D_3_block/2(State_psi_gq_SG_D_3_3b232), d_psi_kq_SG_D_3_block/1(State_psi_gq_SG_D_3_a1641), i_q_SG_D_3_block/1(State_psi_gq_SG_D_3_6f435), T_e_SG_D_3_block/2(State_psi_gq_SG_D_3_f5567), d_psi_kq_SG_D_3_block/3(State_psi_gq_SG_D_3_25fe6)
  Px_2_SG_D_3/1 -> d_Px_3_SG_D_3_block/2(State_Px_2_SG_D_3_6ab48), d_Px_2_SG_D_3_block/1(State_Px_2_SG_D_3_e4ce9), d_Px_3_SG_D_3_block/3(State_Px_2_SG_D_3_b9577)
  psi_q_SG_D_3/1 -> d_psi_q_SG_D_3_block/3(State_psi_q_SG_D_3_df188), d_psi_gq_SG_D_3_block/6(State_psi_q_SG_D_3_1c866), d_psi_kq_SG_D_3_block/5(State_psi_q_SG_D_3_91d06), d_w_SG_D_3_block/6(State_psi_q_SG_D_3_be05f), d_psi_d_SG_D_3_block/8(State_psi_q_SG_D_3_2a9ae), d_V_f_SG_D_3_block/7(State_psi_q_SG_D_3_7abe7), i_d_SG_D_3_block/3(State_psi_q_SG_D_3_0448a), T_e_SG_D_3_block/4(State_psi_q_SG_D_3_e157f), d_w_SG_D_3_block/7(State_psi_q_SG_D_3_3cf4a), i_q_SG_D_3_block/3(State_psi_q_SG_D_3_d128a), d_psi_gq_SG_D_3_block/9(State_psi_q_SG_D_3_e7378), d_V_f_SG_D_3_block/11(State_psi_q_SG_D_3_24c47), T_e_SG_D_3_block/5(State_psi_q_SG_D_3_b3ce3)
  psi_d_SG_D_3/1 -> d_psi_fd_SG_D_3_block/6(State_psi_d_SG_D_3_b2294), d_psi_fd_SG_D_3_block/9(State_psi_d_SG_D_3_a29f0), d_psi_d_SG_D_3_block/2(State_psi_d_SG_D_3_921ca), d_psi_q_SG_D_3_block/8(State_psi_d_SG_D_3_6d66b), d_psi_1d_SG_D_3_block/4(State_psi_d_SG_D_3_a70b8), d_V_f_SG_D_3_block/5(State_psi_d_SG_D_3_0d4e4), d_V_f_SG_D_3_block/12(State_psi_d_SG_D_3_c49cc), d_w_SG_D_3_block/9(State_psi_d_SG_D_3_7b9ed), d_w_SG_D_3_block/3(State_psi_d_SG_D_3_3a32b), i_d_SG_D_3_block/6(State_psi_d_SG_D_3_23dc4), i_q_SG_D_3_block/6(State_psi_d_SG_D_3_56c73), T_e_SG_D_3_block/1(State_psi_d_SG_D_3_e6750), T_e_SG_D_3_block/7(State_psi_d_SG_D_3_a51a8)
  psi_kq_SG_D_3/1 -> d_psi_q_SG_D_3_block/2(State_psi_kq_SG_D_3_0e323), d_psi_gq_SG_D_3_block/3(State_psi_kq_SG_D_3_d7fb5), d_psi_gq_SG_D_3_block/5(State_psi_kq_SG_D_3_5721c), d_psi_gq_SG_D_3_block/8(State_psi_kq_SG_D_3_b0db0), d_psi_kq_SG_D_3_block/2(State_psi_kq_SG_D_3_4633d), d_V_f_SG_D_3_block/10(State_psi_kq_SG_D_3_1ae5a), i_d_SG_D_3_block/2(State_psi_kq_SG_D_3_36d89), i_q_SG_D_3_block/2(State_psi_kq_SG_D_3_72e73), T_e_SG_D_3_block/3(State_psi_kq_SG_D_3_1726a), d_w_SG_D_3_block/5(State_psi_kq_SG_D_3_3748c), d_psi_kq_SG_D_3_block/4(State_psi_kq_SG_D_3_8378f)
  d_psi_kq_SG_D_3_block/1(Blockout_d_psi_kq_SG_D_3_c5bf2) -> psi_kq_SG_D_3/1
  psi_1d_SG_D_3/1 -> d_psi_fd_SG_D_3_block/3(State_psi_1d_SG_D_3_aac28), d_psi_fd_SG_D_3_block/8(State_psi_1d_SG_D_3_845cf), d_psi_d_SG_D_3_block/1(State_psi_1d_SG_D_3_a4437), d_psi_1d_SG_D_3_block/1(State_psi_1d_SG_D_3_8bb29), d_w_SG_D_3_block/8(State_psi_1d_SG_D_3_8c18d), d_V_f_SG_D_3_block/4(State_psi_1d_SG_D_3_b90bf), d_psi_fd_SG_D_3_block/5(State_psi_1d_SG_D_3_07a55), d_psi_1d_SG_D_3_block/3(State_psi_1d_SG_D_3_111f5), i_d_SG_D_3_block/5(State_psi_1d_SG_D_3_0bb66), i_q_SG_D_3_block/5(State_psi_1d_SG_D_3_07363), T_e_SG_D_3_block/6(State_psi_1d_SG_D_3_cd401)
  T_m_SG_D_3/1 -> d_T_m_SG_D_3_block/2(State_T_m_SG_D_3_dcae6), d_w_SG_D_3_block/2(State_T_m_SG_D_3_94420)
  d_R_f_SG_D_3_block/1(Blockout_d_R_f_SG_D_3_2f717) -> R_f_SG_D_3/1
  d_psi_q_SG_D_3_block/1(Blockout_d_psi_q_SG_D_3_0049f) -> psi_q_SG_D_3/1
  d_psi_d_SG_D_3_block/1(Blockout_d_psi_d_SG_D_3_d08c6) -> psi_d_SG_D_3/1
  i_d_SG_D_3_block/1(Blockout_i_d_SG_D_3_0a1a0) -> i_d_SG_D_3/1
  i_q_SG_D_3_block/1(Blockout_i_q_SG_D_3_b9349) -> i_q_SG_D_3/1
  d_psi_gq_SG_D_3_block/1(Blockout_d_psi_gq_SG_D_3_3141c) -> psi_gq_SG_D_3/1
  d_V_f_SG_D_3_block/1(Blockout_d_V_f_SG_D_3_c2e63) -> V_f_SG_D_3/1
  theta_SG_D_3_out_block/1(Blockout_theta_SG_D_3_out_690e3) -> theta_SG_D_3_out/1
  d_psi_1d_SG_D_3_block/1(Blockout_d_psi_1d_SG_D_3_f73a2) -> psi_1d_SG_D_3/1
  T_e_SG_D_3_block/1(Blockout_T_e_SG_D_3_6da4d) -> T_e_SG_D_3/1
  V_f_SG_D_3/1 -> d_V_f_SG_D_3_block/14(State_V_f_SG_D_3_1e7e8), d_E_fd_SG_D_3_block/2(State_V_f_SG_D_3_e8d17)
  Px_3_SG_D_3/1 -> d_V_f_SG_D_3_block/3(State_Px_3_SG_D_3_79789), d_Px_3_SG_D_3_block/1(State_Px_3_SG_D_3_99451)
  d_E_fd_SG_D_3_block/1(Blockout_d_E_fd_SG_D_3_4d917) -> E_fd_SG_D_3/1
  E_fd_SG_D_3/1 -> d_E_fd_SG_D_3_block/1(State_E_fd_SG_D_3_97dd1), d_R_f_SG_D_3_block/1(State_E_fd_SG_D_3_decea), d_psi_fd_SG_D_3_block/1(State_E_fd_SG_D_3_0f771), d_V_f_SG_D_3_block/1(State_E_fd_SG_D_3_0bbdc)
  d_psi_fd_SG_D_3_block/1(Blockout_d_psi_fd_SG_D_3_52489) -> psi_fd_SG_D_3/1

== system case2/AC_1/d_id_line_1_4_block ==
  note: d_id_line_1_4 in case2
      | $376.991118430775\,\mathrm{iq}_{\mathrm{line},1,4}+6679.98156752849\,\mathrm{vd}_{\mathrm{bus},1}-6679.98156752849\,\mathrm{vd}_{\mathrm{bus},4}$
      | Automatically generated on 2025-10-31 18:56:50 .
  State_iq_line_1_4_436b3 : Inport
  State_vd_bus_1_02b8d : Inport  Port=2
  State_vd_bus_4_b081e : Inport  Port=3
  Add_65dc1 : Sum
  Constant_376.991118430775_2289a : Constant  Value=376.991118430775
  Constant_6679.98156752849_8e63a : Constant  Value=6679.98156752849
  Constant_6679.98156752849_a7244 : Constant  Value=6679.98156752849
  Product_bda44 : Product
  Product_c7cd6 : Product
  Product_e50e9 : Product
  Subtract_c52be : Sum  Inputs=+-
  Blockout_d_id_line_1_4_0ab3f : Outport
  wires:
  Constant_376.991118430775_2289a/1 -> Product_c7cd6/1
  Product_bda44/1 -> Add_65dc1/2
  State_iq_line_1_4_436b3/1 -> Product_c7cd6/2
  Subtract_c52be/1 -> Blockout_d_id_line_1_4_0ab3f/1
  Constant_6679.98156752849_8e63a/1 -> Product_bda44/1
  Product_c7cd6/1 -> Add_65dc1/1
  State_vd_bus_1_02b8d/1 -> Product_bda44/2
  Constant_6679.98156752849_a7244/1 -> Product_e50e9/1
  State_vd_bus_4_b081e/1 -> Product_e50e9/2
  Add_65dc1/1 -> Subtract_c52be/1
  Product_e50e9/1 -> Subtract_c52be/2

== system case2/AC_1/d_id_line_3_6_block ==
  note: d_id_line_3_6 in case2
      | $376.991118430775\,\mathrm{iq}_{\mathrm{line},3,6}+6565.98870801435\,\mathrm{vd}_{\mathrm{bus},3}-6565.98870801435\,\mathrm{vd}_{\mathrm{bus},6}$
      | Automatically generated on 2025-10-31 18:56:57 .
  State_iq_line_3_6_4c99f : Inport
  State_vd_bus_3_54849 : Inport  Port=2
  State_vd_bus_6_1884c : Inport  Port=3
  Add_043e6 : Sum
  Constant_376.991118430775_1a120 : Constant  Value=376.991118430775
  Constant_6565.98870801435_bbad6 : Constant  Value=6565.98870801435
  Constant_6565.98870801435_c5125 : Constant  Value=6565.98870801435
  Product_7771e : Product
  Product_c6fe1 : Product
  Product_d897e : Product
  Subtract_caec5 : Sum  Inputs=+-
  Blockout_d_id_line_3_6_a1287 : Outport
  wires:
  State_vd_bus_3_54849/1 -> Product_7771e/2
  Constant_376.991118430775_1a120/1 -> Product_c6fe1/1
  Product_7771e/1 -> Add_043e6/2
  State_iq_line_3_6_4c99f/1 -> Product_c6fe1/2
  Constant_6565.98870801435_bbad6/1 -> Product_7771e/1
  Product_c6fe1/1 -> Add_043e6/1
  Constant_6565.98870801435_c5125/1 -> Product_d897e/1
  State_vd_bus_6_1884c/1 -> Product_d897e/2
  Add_043e6/1 -> Subtract_caec5/1
  Product_d897e/1 -> Subtract_caec5/2
  Subtract_caec5/1 -> Blockout_d_id_line_3_6_a1287/1

== system case2/AC_1/d_id_line_4_5_block ==
  note: d_id_line_4_5 in case2
      | $376.991118430775\,\mathrm{iq}_{\mathrm{line},4,5}-67.4428209618997\,\mathrm{id}_{\mathrm{line},4,5}+4182.24932923523\,\mathrm{vd}_{\mathrm{bus},4}-4182.24932923523\,\mathrm{vd}_{\mathrm{bus},5}$
      | Automatically generated on 2025-10-31 18:56:52 .
  State_id_line_4_5_63ee7 : Inport
  State_iq_line_4_5_db19e : Inport  Port=2
  State_vd_bus_4_38f30 : Inport  Port=3
  State_vd_bus_5_ef8f6 : Inport  Port=4
  Add_2af66 : Sum
  Add_9acd2 : Sum
  Constant_-67.4428209618997_cfa87 : Constant  Value=-67.4428209618997
  Constant_376.991118430775_aa676 : Constant  Value=376.991118430775
  Constant_4182.24932923523_255c8 : Constant  Value=4182.24932923523
  Constant_4182.24932923523_7487c : Constant  Value=4182.24932923523
  Product_4c003 : Product
  Product_66f0f : Product
  Product_ceea4 : Product
  Product_dd33e : Product
  Subtract_b695a : Sum  Inputs=+-
  Blockout_d_id_line_4_5_ba811 : Outport
  wires:
  Constant_-67.4428209618997_cfa87/1 -> Product_66f0f/1
  Product_ceea4/1 -> Add_2af66/2
  State_id_line_4_5_63ee7/1 -> Product_66f0f/2
  Constant_376.991118430775_aa676/1 -> Product_ceea4/1
  State_iq_line_4_5_db19e/1 -> Product_ceea4/2
  Product_66f0f/1 -> Add_2af66/1
  Constant_4182.24932923523_7487c/1 -> Product_dd33e/1
  State_vd_bus_4_38f30/1 -> Product_dd33e/2
  Add_2af66/1 -> Add_9acd2/1
  Product_dd33e/1 -> Add_9acd2/2
  Constant_4182.24932923523_255c8/1 -> Product_4c003/1
  State_vd_bus_5_ef8f6/1 -> Product_4c003/2
  Add_9acd2/1 -> Subtract_b695a/1
  Product_4c003/1 -> Subtract_b695a/2
  Subtract_b695a/1 -> Blockout_d_id_line_4_5_ba811/1

== system case2/AC_1/d_id_line_5_6_block ==
  note: d_id_line_5_6 in case2
      | $376.991118430775\,\mathrm{iq}_{\mathrm{line},5,6}-83.7317791042547\,\mathrm{id}_{\mathrm{line},5,6}+2263.33493111553\,\mathrm{vd}_{\mathrm{bus},5}-2263.33493111553\,\mathrm{vd}_{\mathrm{bus},6}$
      | Automatically generated on 2025-10-31 18:56:54 .
  State_id_line_5_6_54864 : Inport
  State_iq_line_5_6_98e26 : Inport  Port=2
  State_vd_bus_5_724a2 : Inport  Port=3
  State_vd_bus_6_a9a0a : Inport  Port=4
  Add_430fd : Sum
  Add_5ec87 : Sum
  Constant_-83.7317791042547_bbccd : Constant  Value=-83.7317791042547
  Constant_2263.33493111553_152d0 : Constant  Value=2263.33493111553
  Constant_2263.33493111553_b1a70 : Constant  Value=2263.33493111553
  Constant_376.991118430775_d9f90 : Constant  Value=376.991118430775
  Product_233fd : Product
  Product_32012 : Product
  Product_51a4e : Product
  Product_cf85b : Product
  Subtract_8e0ee : Sum  Inputs=+-
  Blockout_d_id_line_5_6_f183f : Outport
  wires:
  Constant_-83.7317791042547_bbccd/1 -> Product_233fd/1
  Product_51a4e/1 -> Add_5ec87/2
  State_id_line_5_6_54864/1 -> Product_233fd/2
  Constant_376.991118430775_d9f90/1 -> Product_51a4e/1
  Product_233fd/1 -> Add_5ec87/1
  State_iq_line_5_6_98e26/1 -> Product_51a4e/2
  Constant_2263.33493111553_b1a70/1 -> Product_32012/1
  Product_cf85b/1 -> Subtract_8e0ee/2
  State_vd_bus_5_724a2/1 -> Product_32012/2
  Add_5ec87/1 -> Add_430fd/1
  Product_32012/1 -> Add_430fd/2
  Constant_2263.33493111553_152d0/1 -> Product_cf85b/1
  State_vd_bus_6_a9a0a/1 -> Product_cf85b/2
  Add_430fd/1 -> Subtract_8e0ee/1
  Subtract_8e0ee/1 -> Blockout_d_id_line_5_6_f183f/1

== system case2/AC_1/d_id_line_6_7_block ==
  note: d_id_line_6_7 in case2
      | $376.991118430775\,\mathrm{iq}_{\mathrm{line},6,7}-43.0884689478804\,\mathrm{id}_{\mathrm{line},6,7}+3817.13232430199\,\mathrm{vd}_{\mathrm{bus},6}-3817.13232430199\,\mathrm{vd}_{\mathrm{bus},7}$
      | Automatically generated on 2025-10-31 18:56:59 .
  State_id_line_6_7_5f97c : Inport
  State_iq_line_6_7_b228d : Inport  Port=2
  State_vd_bus_6_7ad19 : Inport  Port=3
  State_vd_bus_7_c0c3c : Inport  Port=4
  Add_fb80f : Sum
  Add_ff7ab : Sum
  Constant_-43.0884689478804_e1c7c : Constant  Value=-43.0884689478804
  Constant_376.991118430775_fc0c6 : Constant  Value=376.991118430775
  Constant_3817.13232430199_5373f : Constant  Value=3817.13232430199
  Constant_3817.13232430199_9afde : Constant  Value=3817.13232430199
  Product_54205 : Product
  Product_89499 : Product
  Product_a8797 : Product
  Product_fbdb6 : Product
  Subtract_fea24 : Sum  Inputs=+-
  Blockout_d_id_line_6_7_9dd44 : Outport
  wires:
  Constant_-43.0884689478804_e1c7c/1 -> Product_fbdb6/1
  Product_89499/1 -> Add_ff7ab/2
  State_id_line_6_7_5f97c/1 -> Product_fbdb6/2
  Constant_376.991118430775_fc0c6/1 -> Product_89499/1
  State_iq_line_6_7_b228d/1 -> Product_89499/2
  Product_fbdb6/1 -> Add_ff7ab/1
  Constant_3817.13232430199_5373f/1 -> Product_54205/1
  State_vd_bus_6_7ad19/1 -> Product_54205/2
  Add_ff7ab/1 -> Add_fb80f/1
  Product_54205/1 -> Add_fb80f/2
  Constant_3817.13232430199_9afde/1 -> Product_a8797/1
  State_vd_bus_7_c0c3c/1 -> Product_a8797/2
  Add_fb80f/1 -> Subtract_fea24/1
  Product_a8797/1 -> Subtract_fea24/2
  Subtract_fea24/1 -> Blockout_d_id_line_6_7_9dd44/1

== system case2/AC_1/d_id_line_7_8_block ==
  note: d_id_line_7_8 in case2
      | $376.991118430775\,\mathrm{iq}_{\mathrm{line},7,8}-43.0884689478804\,\mathrm{id}_{\mathrm{line},7,8}+5343.98525402279\,\mathrm{vd}_{\mathrm{bus},7}-5343.98525402279\,\mathrm{vd}_{\mathrm{bus},8}$
      | Automatically generated on 2025-10-31 18:57:02 .
  State_id_line_7_8_397f6 : Inport
  State_iq_line_7_8_44268 : Inport  Port=2
  State_vd_bus_7_f48ac : Inport  Port=3
  State_vd_bus_8_1c270 : Inport  Port=4
  Add_9f7c7 : Sum
  Add_fadb5 : Sum
  Constant_-43.0884689478804_00ebd : Constant  Value=-43.0884689478804
  Constant_376.991118430775_baa1f : Constant  Value=376.991118430775
  Constant_5343.98525402279_0da11 : Constant  Value=5343.98525402279
  Constant_5343.98525402279_7f825 : Constant  Value=5343.98525402279
  Product_1a31b : Product
  Product_5bd45 : Product
  Product_e892b : Product
  Product_fe339 : Product
  Subtract_78b28 : Sum  Inputs=+-
  Blockout_d_id_line_7_8_bc37b : Outport
  wires:
  Constant_-43.0884689478804_00ebd/1 -> Product_1a31b/1
  Product_fe339/1 -> Add_fadb5/2
  State_id_line_7_8_397f6/1 -> Product_1a31b/2
  Constant_376.991118430775_baa1f/1 -> Product_fe339/1
  Product_1a31b/1 -> Add_fadb5/1
  State_iq_line_7_8_44268/1 -> Product_fe339/2
  Constant_5343.98525402279_0da11/1 -> Product_5bd45/1
  State_vd_bus_7_f48ac/1 -> Product_5bd45/2
  Add_fadb5/1 -> Add_9f7c7/1
  Product_5bd45/1 -> Add_9f7c7/2
  Constant_5343.98525402279_7f825/1 -> Product_e892b/1
  State_vd_bus_8_1c270/1 -> Product_e892b/2
  Add_9f7c7/1 -> Subtract_78b28/1
  Product_e892b/1 -> Subtract_78b28/2
  Subtract_78b28/1 -> Blockout_d_id_line_7_8_bc37b/1

== system case2/AC_1/d_id_line_8_2_block ==
  note: d_id_line_8_2 in case2
      | $376.991118430775\,\mathrm{iq}_{\mathrm{line},8,2}-6156.27101263426\,\mathrm{vd}_{\mathrm{bus},2}+6156.27101263426\,\mathrm{vd}_{\mathrm{bus},8}$
      | Automatically generated on 2025-10-31 18:57:04 .
  State_iq_line_8_2_cd298 : Inport
  State_vd_bus_2_94e9c : Inport  Port=2
  State_vd_bus_8_dfb0e : Inport  Port=3
  Add_2fa6b : Sum
  Constant_376.991118430775_4c349 : Constant  Value=376.991118430775
  Constant_6156.27101263426_b4394 : Constant  Value=6156.27101263426
  Constant_6156.27101263426_dc764 : Constant  Value=6156.27101263426
  Product_a825d : Product
  Product_b8c90 : Product
  Product_dfddc : Product
  Subtract_97d27 : Sum  Inputs=+-
  Blockout_d_id_line_8_2_9ff87 : Outport
  wires:
  State_vd_bus_2_94e9c/1 -> Product_dfddc/2
  Constant_376.991118430775_4c349/1 -> Product_a825d/1
  Product_dfddc/1 -> Subtract_97d27/2
  State_iq_line_8_2_cd298/1 -> Product_a825d/2
  Constant_6156.27101263426_dc764/1 -> Product_dfddc/1
  Product_a825d/1 -> Subtract_97d27/1
  Constant_6156.27101263426_b4394/1 -> Product_b8c90/1
  State_vd_bus_8_dfb0e/1 -> Product_b8c90/2
  Subtract_97d27/1 -> Add_2fa6b/1
  Product_b8c90/1 -> Add_2fa6b/2
  Add_2fa6b/1 -> Blockout_d_id_line_8_2_9ff87/1

== system case2/AC_1/d_id_line_8_9_block ==
  note: d_id_line_8_9 in case2
      | $376.991118430775\,\mathrm{iq}_{\mathrm{line},8,9}-72.54353851364\,\mathrm{id}_{\mathrm{line},8,9}+2389.85675956299\,\mathrm{vd}_{\mathrm{bus},8}-2389.85675956299\,\mathrm{vd}_{\mathrm{bus},9}$
      | Automatically generated on 2025-10-31 18:57:06 .
  State_id_line_8_9_36022 : Inport
  State_iq_line_8_9_f99c7 : Inport  Port=2
  State_vd_bus_8_d11ac : Inport  Port=3
  State_vd_bus_9_a61c1 : Inport  Port=4
  Add_6c197 : Sum
  Add_e81a8 : Sum
  Constant_-72.54353851364_5d8eb : Constant  Value=-72.54353851364
  Constant_2389.85675956299_0f732 : Constant  Value=2389.85675956299
  Constant_2389.85675956299_443ed : Constant  Value=2389.85675956299
  Constant_376.991118430775_50d22 : Constant  Value=376.991118430775
  Product_32b6c : Product
  Product_581d8 : Product
  Product_cae4f : Product
  Product_d5395 : Product
  Subtract_6ffb1 : Sum  Inputs=+-
  Blockout_d_id_line_8_9_70ad0 : Outport
  wires:
  Constant_-72.54353851364_5d8eb/1 -> Product_32b6c/1
  Product_581d8/1 -> Add_e81a8/2
  State_id_line_8_9_36022/1 -> Product_32b6c/2
  Constant_376.991118430775_50d22/1 -> Product_581d8/1
  State_iq_line_8_9_f99c7/1 -> Product_581d8/2
  Product_32b6c/1 -> Add_e81a8/1
  Constant_2389.85675956299_443ed/1 -> Product_d5395/1
  State_vd_bus_8_d11ac/1 -> Product_d5395/2
  Add_e81a8/1 -> Add_6c197/1
  Product_d5395/1 -> Add_6c197/2
  Constant_2389.85675956299_0f732/1 -> Product_cae4f/1
  State_vd_bus_9_a61c1/1 -> Product_cae4f/2
  Add_6c197/1 -> Subtract_6ffb1/1
  Product_cae4f/1 -> Subtract_6ffb1/2
  Subtract_6ffb1/1 -> Blockout_d_id_line_8_9_70ad0/1

== system case2/AC_1/d_id_line_9_4_block ==
  note: d_id_line_9_4 in case2
      | $376.991118430775\,\mathrm{iq}_{\mathrm{line},9,4}-42.9393738996178\,\mathrm{id}_{\mathrm{line},9,4}-4526.66986223107\,\mathrm{vd}_{\mathrm{bus},4}+4526.66986223107\,\mathrm{vd}_{\mathrm{bus},9}$
      | Automatically generated on 2025-10-31 18:57:09 .
  State_id_line_9_4_78432 : Inport
  State_iq_line_9_4_7582d : Inport  Port=2
  State_vd_bus_4_3cbcb : Inport  Port=3
  State_vd_bus_9_e3f3e : Inport  Port=4
  Add_64000 : Sum
  Add_a9af6 : Sum
  Constant_-42.9393738996178_19c1b : Constant  Value=-42.9393738996178
  Constant_376.991118430775_68ba9 : Constant  Value=376.991118430775
  Constant_4526.66986223107_9064d : Constant  Value=4526.66986223107
  Constant_4526.66986223107_d8c22 : Constant  Value=4526.66986223107
  Product_4b428 : Product
  Product_4f43b : Product
  Product_5e246 : Product
  Product_99379 : Product
  Subtract_fa632 : Sum  Inputs=+-
  Blockout_d_id_line_9_4_e7536 : Outport
  wires:
  Constant_-42.9393738996178_19c1b/1 -> Product_5e246/1
  Product_4b428/1 -> Add_a9af6/2
  State_id_line_9_4_78432/1 -> Product_5e246/2
  Constant_376.991118430775_68ba9/1 -> Product_4b428/1
  Product_5e246/1 -> Add_a9af6/1
  State_iq_line_9_4_7582d/1 -> Product_4b428/2
  Constant_4526.66986223107_9064d/1 -> Product_99379/1
  State_vd_bus_4_3cbcb/1 -> Product_99379/2
  Add_a9af6/1 -> Subtract_fa632/1
  Product_99379/1 -> Subtract_fa632/2
  Constant_4526.66986223107_d8c22/1 -> Product_4f43b/1
  Subtract_fa632/1 -> Add_64000/1
  State_vd_bus_9_e3f3e/1 -> Product_4f43b/2
  Product_4f43b/1 -> Add_64000/2
  Add_64000/1 -> Blockout_d_id_line_9_4_e7536/1

== system case2/AC_1/d_id_load_5_block ==
  note: d_id_load_5 in case2
      | $376.991118430775\,\mathrm{iq}_{\mathrm{load},5}-1149.14023057989\,\mathrm{id}_{\mathrm{load},5}+1237.92955189927\,\mathrm{vd}_{\mathrm{bus},5}$
      | Automatically generated on 2025-10-31 18:56:44 .
  State_id_load_5_57de7 : Inport
  State_iq_load_5_85fa6 : Inport  Port=2
  State_vd_bus_5_7c4d9 : Inport  Port=3
  Add_1b468 : Sum
  Add_2251e : Sum
  Constant_-1149.14023057989_ca5bb : Constant  Value=-1149.14023057989
  Constant_1237.92955189927_f3fa3 : Constant  Value=1237.92955189927
  Constant_376.991118430775_4281f : Constant  Value=376.991118430775
  Product_4c971 : Product
  Product_79b83 : Product
  Product_9a393 : Product
  Blockout_d_id_load_5_8438f : Outport
  wires:
  Constant_-1149.14023057989_ca5bb/1 -> Product_4c971/1
  Product_79b83/1 -> Add_1b468/2
  State_id_load_5_57de7/1 -> Product_4c971/2
  Constant_376.991118430775_4281f/1 -> Product_79b83/1
  Product_9a393/1 -> Add_2251e/2
  State_iq_load_5_85fa6/1 -> Product_79b83/2
  Product_4c971/1 -> Add_1b468/1
  Constant_1237.92955189927_f3fa3/1 -> Product_9a393/1
  State_vd_bus_5_7c4d9/1 -> Product_9a393/2
  Add_1b468/1 -> Add_2251e/1
  Add_2251e/1 -> Blockout_d_id_load_5_8438f/1
